simulink library "MyLibrary"  (R2018b)
settings: Solver=VariableStepAuto  StartTime=0.0  StopTime=10.0  RelTol=1e-3
undefined symbols (not defined in the file or in its folder): gcbh, sps_rtmsupport
libraries: spsUniversalBridgeModel x1
settings Model: Creator=ThinkPad  LastModifiedBy=ThinkPad

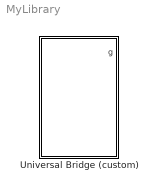
== system MyLibrary ==
  Universal Bridge (custom) : Subsystem  DialogController=POWERSYS.PowerSysDialog  LoadFcn=sps_rtmsupport('LoadFcn',gcbh);  StartFcn=sps_rtmsupport('StartFcn',gcbh);  StopFcn=sps_rtmsupport('StopFcn',gcbh);  mask(Universal Bridge){Arms=3, SnubberResistance=1e5, SnubberCapacitance=inf, Device=IGBT / Diodes, Ron=1e-3, Lon=0, ForwardVoltages=[  3  2  ], ForwardVoltage=0, GTOparameters=[ 10e-6 , 20e-6 ], IGBTparameters=[ 1e-6 , 2e-6 ], Measurements=All voltages and currents, Measurements_2=None, converterType=Rectifier}
      mask prompts: Arms "Number of bridge arms:"; SnubberResistance "Snubber resistance Rs (Ohms)"; SnubberCapacitance "Snubber capacitance Cs (F)"; Device "Power Electronic device"; Ron "Ron (Ohms)"; Lon "Lon (H)"; ForwardVoltages "Forward voltages  [ Device Vf(V) , Diode Vfd(V)]"; ForwardVoltage "Forward voltage Vf (V)"; GTOparameters "[  Tf (s) , Tt (s)  ]"; IGBTparameters "[  Tf (s) , Tt (s)  ]"; Measurements_2 "Measurements"; converterType "Converter type:"
      settings: CopyFcn=sps_rtmsupport('CopyFcn',gcbh); powericon('SwitchesCopyFcn','Universal Bridge',gcb)  DeleteFcn=sps_rtmsupport('DeleteFcn',gcbh);  UndoDeleteFcn=sps_rtmsupport('UndoDeleteFcn',gcbh);  ModelCloseFcn=sps_rtmsupport('ModelCloseFcn',gcbh);  PreSaveFcn=sps_rtmsupport('PreSaveFcn',gcbh);  PostSaveFcn=sps_rtmsupport('PostSaveFcn',gcbh);  NameChangeFcn=sps_rtmsupport('NameChangeFcn',gcbh);  PreCopyFcn=sps_rtmsupport('PreCopyFcn',gcbh);  OpenFcn=sps_rtmsupport('OpenFcn',gcbh, [1 4 11 12 13]);  CloseFcn=sps_rtmsupport('CloseFcn',gcbh);  PreDeleteFcn=sps_rtmsupport('PreDeleteFcn',gcbh);
      mask TypeOptions Arms: 1 | 2 | 3
      mask Callback Arms: powericon('UniversalBridgeCback',gcb);
      mask TypeOptions Device: Diodes | Thyristors | GTO / Diodes | MOSFET / Diodes | IGBT / Diodes | Ideal Switches | Switching-function based VSC | Average-model based VSC
      mask Callback Device: powericon('UniversalBridgeCback',gcb);
      mask TypeOptions Measurements: None | Device voltages | Device currents | UAB UBC UCA UDC voltages | All voltages and currents
      mask TypeOptions Measurements_2: None | Voltages | Currents | Voltages and Currents
      mask TypeOptions converterType: Rectifier | Inverter

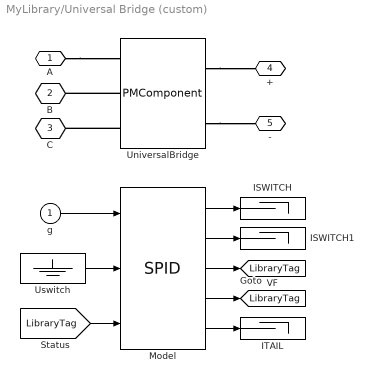
== system MyLibrary/Universal Bridge (custom) ==
  g : Inport
  ISWITCH : Terminator
  ISWITCH1 : Terminator
  ITAIL : Terminator
  Model : spsUniversalBridgeModel/SPID  SystemSampleTime=-1
  UniversalBridge : PMComponent  PhysicalDomain=powersysdomain  LeftPortType=p1  RightPortType=p1  LConnTagsString=A|B|C  RConnTagsString=+|-  mask(InnerPowersysBlock){}
      mask Display: disp('SPS internal use\nDo not delete')
  Uswitch : Ground
  A : PMIOPort  Side=Left
  B : PMIOPort  Port=2  Side=Left
  C : PMIOPort  Port=3  Side=Left
  + : PMIOPort  Port=4  Side=Right
  - : PMIOPort  Port=5  Side=Right
  tag scope: LibraryTag=global
  wires:
  Model/2 -> ISWITCH1/1
  Model/1 -> ISWITCH/1
  Model/5 -> ITAIL/1
  Model/3 -> [LibraryTag]
  Model/4 -> [LibraryTag]
  [LibraryTag] -> Model/3
  Uswitch/1 -> Model/2
  g/1 -> Model/1
  connections:
  A/RConn1 -- UniversalBridge/LConn1
  UniversalBridge/RConn1 -- +/RConn1
  UniversalBridge/RConn2 -- -/RConn1
  UniversalBridge/LConn2 -- B/RConn1
  UniversalBridge/LConn3 -- C/RConn1
